simulink model "lab3"  (R2020b)
settings: Solver=VariableStepAuto  StartTime=0.0  StopTime=10.0  RelTol=1e-3
model workspace (MAT data in the model file):
  a = Simulink.Parameter
  a.Value = 1
  a.DataType = 'auto'
  a.Dimensions = [1 1]
  b = Simulink.Parameter
  b.Value = 0.5792
  b.DataType = 'auto'
  b.Dimensions = [1 1]
  c = Simulink.Parameter
  c.Value = 0.1584
  c.DataType = 'auto'
  c.Dimensions = [1 1]
  d = Simulink.Parameter
  d.Value = -0.5792
  d.DataType = 'auto'
  d.Dimensions = [1 1]
settings Model: Creator=sushma  LastModifiedBy=sushma

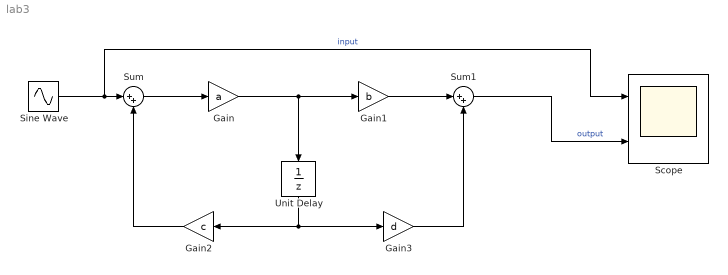
== system lab3 ==
  Gain : Gain  Gain=a
  Gain1 : Gain  Gain=b
  Gain2 : Gain  Gain=c
  Gain3 : Gain  Gain=d
  Scope : Scope  NumInputPorts=2
  Sine Wave : Sin  Frequency=6500  SampleTime=0
  Sum : Sum  Inputs=|++
  Sum1 : Sum  Inputs=|++
  Unit Delay : UnitDelay  SampleTime=-1  HasFrameUpgradeWarning=on
  wires:
  Sum/1 -> Gain/1
  Gain/1 -> Unit Delay/1, Gain1/1
  Gain1/1 -> Sum1/1
  Unit Delay/1 -> Gain2/1, Gain3/1
  Gain2/1 -> Sum/2
  Gain3/1 -> Sum1/2
  Sum1/1 -> Scope/2  "output"
  Sine Wave/1 -> Scope/1, Sum/1  "input"
